simulink model "OneRobot_proporcional"  (R2021b)
settings: Solver=FixedStepDiscrete  StartTime=0.0  StopTime=t_sim  FixedStep=0.01  RelTol=1e-3  EnableMultiTasking=on
model workspace (MAT data in the model file):
  rampa = 1
values from neighbouring files (symbols this model uses):
  x = x-0.1    [movimiento.m]
  y = y-0.1    [movimiento.m]
undefined symbols (not defined in the file or in its folder): a, Angular, Linear, rx1, ry1
libraries: robotlib x4, robotcorelib x1, robotalgslib x1
settings Model: PacingRate=0.450000  Creator=The MathWorks, Inc.  LastModifiedBy=Cinthy
settings SolverCC: ConcurrentTasks=on  AlgebraicLoopSolver=TrustRegion  AutoInsertRateTranBlk=on
settings DataIOCC: LimitDataPoints=on  SaveFormat=StructureWithTime  ReturnWorkspaceOutputs=off
settings OptimizationCC: BlockReduction=off  EnhancedBackFolding=on  PassReuseOutputArgsAs=Individual arguments  ZeroExternalMemoryAtStartup=off  ZeroInternalMemoryAtStartup=off  MaxStackSize=64  OptimizeBlockOrder=speed  DifferentSizesBufferReuse=on  OptimizationCustomize=off  EfficientTunableParamExpr=on
settings DebuggingCC: SolverPrmCheckMsg=warning  ParameterTunabilityLossMsg=error  SFUnexpectedBacktrackingDiag=warning  SFNoUnconditionalDefaultTransitionDiag=warning  SFExecutionAtInitializationDiag=none  SFMachineParentedDataDiag=warning  ArithmeticOperatorsInVariantConditions=warning
settings HardwareCC: ProdBitPerPointer=32  ProdBitPerSizeT=32  ProdBitPerPtrDiffT=32  ProdLargestAtomicFloat=None  ProdIntDivRoundTo=Undefined  ProdEndianess=Unspecified  ProdWordSize=32  ProdHWDeviceType=Generic->Unspecified (assume 32-bit Generic)  TargetHWDeviceType=Generic->Unspecified (assume 32-bit Generic)
settings ModelReferenceCC: PropagateSignalLabelsOutOfModel=off
settings SFSimCC: SimUseLocalCustomCode=off  MATLABDynamicMemAlloc=off  CustomCodeUndefinedFunction=UseInterfaceOnly  SimTargetLang=C++
settings RTWCC: Description=Embedded Coder  SystemTargetFile=ert.tlc  HardwareBoard=Robot Operating System (ROS)  TLCOptions="-aInlineSetEventsForThisBaseRateFcn=TLC_FALSE -aSuppressMultiTaskScheduler=TLC_FALSE  -aRateBasedStepFcn=0"  TemplateMakefile=ert_default_tmf  RTWUseLocalCustomCode=off  Toolchain=Catkin  TargetLang=C++
settings CodeAppCC: ForceParamTrailComments=on  IgnoreCustomStorageClasses=off  OperatorAnnotations=on  SimulinkDataObjDesc=on  SFDataObjDesc=on  InsertBlockDesc=on
settings ConfigComp: CovMetricSettings=dw  CovSaveCumulativeToWorkspaceVar=on  CovSaveSingleToWorkspaceVar=on  CovExternalEMLEnable=off  CovSFcnEnable=off

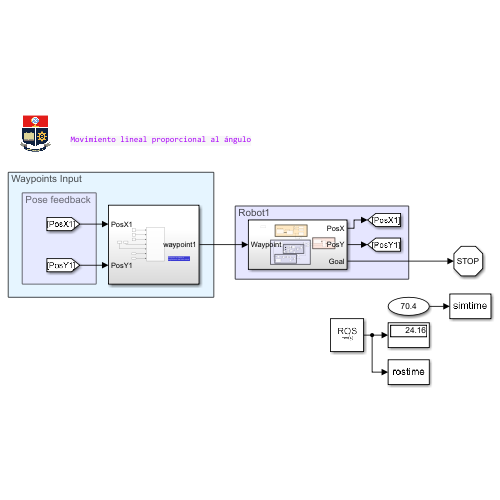
[thumbnail: Simulink's stored preview of the top-level diagram]
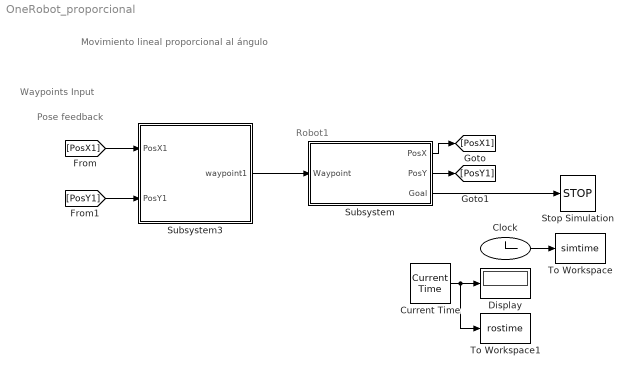
== system OneRobot_proporcional ==
  note: Movimiento lineal proporcional al ángulo
  note: Pose feedback
  note: Robot1
  note: Waypoints Input
  Clock : Clock
  Current Time : robotlib/Current Time  OutputFormat=double  SampleTime=-1  ModelName=OneRobot_proporcional
      settings: SourceProductBaseCode=RR
  Display : Display
  Stop Simulation : Stop
  Subsystem : Subsystem
  Subsystem3 : Subsystem
  To Workspace : ToWorkspace  VariableName=simtime  SampleTime=-1
  To Workspace1 : ToWorkspace  VariableName=rostime  SampleTime=-1
  wires:
  Subsystem/1(PosX) -> [PosX1]
  Subsystem/2(PosY) -> [PosY1]
  Subsystem3/1(waypoint1) -> Subsystem/1(Waypoint)
  Subsystem/3(Goal) -> Stop Simulation/1
  Clock/1 -> To Workspace/1
  [PosX1] -> Subsystem3/1(PosX1)
  [PosY1] -> Subsystem3/2(PosY1)
  Current Time/1 -> To Workspace1/1, Display/1

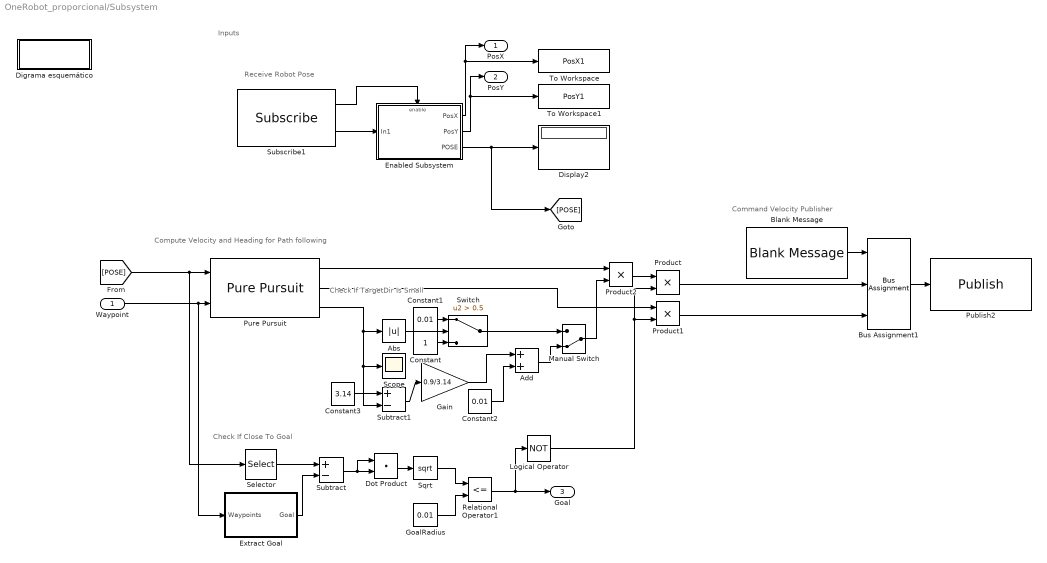
== system OneRobot_proporcional/Subsystem ==
  note: Check If TargetDir Is Small
  note: Compute Velocity and Heading for Path following
  note: Inputs
  note: Receive Robot Pose
  note: Check If Close To Goal
  note: Command Velocity Publisher
  Waypoint : Inport
  " Extract Goal" : MATLAB Function  TreatAsAtomicUnit=on
  Abs : Abs
  Add : Sum
  Blank Message : robotlib/Blank Message  messageClass=Message  entityType=geometry_msgs/Twist  messageType=geometry_msgs/Twist  SampleTime=inf  legacyBusStruct=off
  Bus Assignment1 : BusAssignment  DialogController=Simulink.DDGSource_BusAssignment  AssignedSignals=Linear.X,Angular.Z
  Constant : Constant
  Constant1 : Constant  Value=0.01
  Constant2 : Constant  Value=0.01
  Constant3 : Constant  Value=3.14
  Digrama esquemático : Subsystem
  Display2 : Display
  Dot Product : DotProduct  InputSameDT=on  OutDataTypeStr=Inherit: Inherit via internal rule
  Enabled Subsystem : Subsystem
  Gain : Gain  Gain=0.9/3.14
  GoalRadius : Constant  Value=0.01
  Logical Operator : Logic  Operator=NOT  AllPortsSameDT=off  OutDataTypeStr=boolean
  Manual Switch : ManualSwitch  CurrentSetting=0
  Product : Product
  Product1 : Product
  Product2 : Product
  Publish2 : robotlib/Publish  topicSource=Select from ROS network  topic=/robot1/cmd_vel  messageType=geometry_msgs/Twist  legacyBusStruct=off  messageQueueLength=105
  Pure Pursuit : robotalgslib/Pure Pursuit  DesiredLinearVelocity=0.22  MaxAngularVelocity=2.84  LookaheadDistance=1  TargetDirPort=on  SimulateUsing=Code generation
  Relational Operator1 : RelationalOperator  Operator=<=  OutDataTypeStr=boolean  RndMeth=Simplest
  Scope : Scope
  Selector : Selector  InputPortWidth=3  IndexOptions=Index vector (dialog)  Indices=[1 2]  OutputSizes=1
  Sqrt : Sqrt  SaturateOnIntegerOverflow=on
  Subscribe1 : robotlib/Subscribe  topicSource=Select from ROS network  topic=/robot1/odom  messageType=nav_msgs/Odometry  SampleTime=-1  legacyBusStruct=off  messageQueueLength=51
  Subtract : Sum  Inputs=+-
  Subtract1 : Sum  Inputs=+-
  Switch : Switch  Criteria=u2 > Threshold  Threshold=0.5
  To Workspace : ToWorkspace  VariableName=PosX1  SampleTime=-1
  To Workspace1 : ToWorkspace  VariableName=PosY1  SampleTime=-1
  PosX : Outport
  PosY : Outport  Port=2
  Goal : Outport  Port=3
  wires:
  GoalRadius/1 -> Relational Operator1/2
  Blank Message/1 -> Bus Assignment1/1
  Enabled Subsystem/3(POSE) -> [POSE], Display2/1
  Subtract/1 -> Dot Product/1, Dot Product/2
  Enabled Subsystem/2(PosY) -> PosY/1, To Workspace1/1
  Subscribe1/2 -> Enabled Subsystem/1(In1)
  Pure Pursuit/2 -> Product1/1
  Subscribe1/1 -> Enabled Subsystem/Enable
  Enabled Subsystem/1(PosX) -> PosX/1, To Workspace/1
  Relational Operator1/1 -> Logical Operator/1, Goal/1
  Product/1 -> Bus Assignment1/2
  Bus Assignment1/1 -> Publish2/1
  [POSE] -> Pure Pursuit/1, Selector/1
  Dot Product/1 -> Sqrt/1
  " Extract Goal"/1(Goal) -> Subtract/2
  Selector/1 -> Subtract/1
  Sqrt/1 -> Relational Operator1/1
  Logical Operator/1 -> Product1/2, Product/2
  Product1/1 -> Bus Assignment1/3
  Waypoint/1 -> " Extract Goal"/1(Waypoints), Pure Pursuit/2
  Pure Pursuit/3 -> Subtract1/2, Scope/1, Abs/1
  Constant/1 -> Switch/3
  Constant1/1 -> Switch/1
  Product2/1 -> Product/1
  Abs/1 -> Switch/2
  Pure Pursuit/1 -> Product2/1
  Constant2/1 -> Add/2
  Gain/1 -> Add/1
  Add/1 -> Manual Switch/2
  Manual Switch/1 -> Product2/2
  Switch/1 -> Manual Switch/1
  Constant3/1 -> Subtract1/1
  Subtract1/1 -> Gain/1

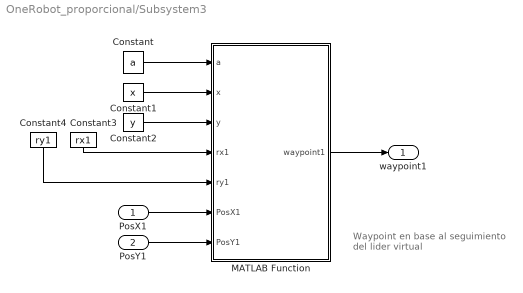
== system OneRobot_proporcional/Subsystem3 ==
  note: Waypoint en base al seguimiento del lider virtual
  PosX1 : Inport
  PosY1 : Inport  Port=2
  Constant : Constant  Value=a
  Constant1 : Constant  Value=x
  Constant2 : Constant  Value=y
  Constant3 : Constant  Value=rx1
  Constant4 : Constant  Value=ry1
  MATLAB Function : MATLAB Function  TreatAsAtomicUnit=on
  waypoint1 : Outport
  wires:
  Constant/1 -> MATLAB Function/1(a)
  Constant2/1 -> MATLAB Function/3(y)
  Constant1/1 -> MATLAB Function/2(x)
  PosX1/1 -> MATLAB Function/6(PosX1)
  MATLAB Function/1(waypoint1) -> waypoint1/1
  PosY1/1 -> MATLAB Function/7(PosY1)
  Constant3/1 -> MATLAB Function/4(rx1)
  Constant4/1 -> MATLAB Function/5(ry1)

== system OneRobot_proporcional/Subsystem/Digrama esquemático ==
  note: Definición de Velocidad lineal y angular
  note: >
  note: _____
  note: Waypoint
  note: |
      | |
      | |
  note: / |
      | [POSE] |
      | \_______|
  note: ______|
  note: Definir mensaje a enviar
  note: Comprobar si llegó a la meta
  note: Condiconamiento de Velocidad lineal
  note: Envio Velocidades al Robot
  note: Control Pure Pursuit
  note: Visualización
  note: Procesamiento de datos
  note: Recibir Pose del Robot
  note: | \
      | | [POSE]
      | |_______/
  note: >
  note: _____
  note: >
  note: _____
  note: _____
  note: >
  note: _____
  note: >
  note: _____
  note: >
  note: >
  note: _____
  note: >
  note: _____
  note: __________________
  note: >
  note: _____
  note: >
  note: _____
  note: >
  note: |
  note: >
  note: ____________________
  note: |
  note: >
  note: ___
  note: |
  note: |
  note: |
  note: ___
  note: _______________________________
  note: >
  note: ___
  note: |
  note: >
  note: _____
  note: |
  note: |
  note: |
  note: |
  note: |
  note: |
  note: |
  note: |
  note: |
  note: |
  note: |
  note: |
  note: |
  note: |
  note: |
  note: |

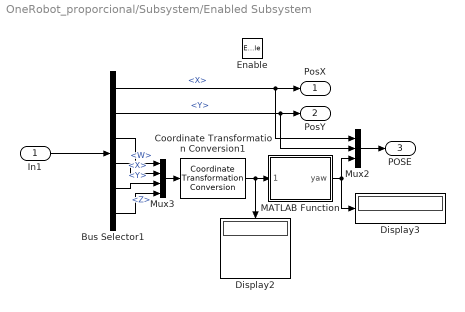
== system OneRobot_proporcional/Subsystem/Enabled Subsystem ==
  In1 : Inport
  Enable : EnablePort
  Bus Selector1 : BusSelector  DialogController=Simulink.DDGSource_BusSelector  OutputSignals=Pose.Pose.Position.X,Pose.Pose.Position.Y,Pose.Pose.Orientation.W,Pose.Pose.Orientation.X,Pose.Pose.Orientation.Y,Pose.Pose.Orientation.Z
  Coordinate Transformation Conversion1 : robotcorelib/Coordinate Transformation Conversion  InputRepresentation=Quaternion  InputEulerSequence=ZYX  ShowTrVecInputPort=on  OutputRepresentation=Euler Angles  OutputEulerSequence=ZYX  ShowTrVecOutputPort=on  SimulateUsing=Interpreted execution
      settings: SourceProductBaseCode=NV,RO,RR,UV
  Display2 : Display
  Display3 : Display
  MATLAB Function : MATLAB Function  TreatAsAtomicUnit=on
  Mux2 : Mux  Inputs=3
  Mux3 : Mux
  PosX : Outport  VectorParamsAs1DForOutWhenUnconnected=off
  PosY : Outport  Port=2  VectorParamsAs1DForOutWhenUnconnected=off
  POSE : Outport  Port=3
  wires:
  Bus Selector1/5 -> Mux3/3  "<Y>"
  Bus Selector1/1 -> PosX/1, Mux2/1  "<X>"
  Bus Selector1/3 -> Mux3/1  "<W>"
  Mux2/1 -> POSE/1
  In1/1 -> Bus Selector1/1
  Coordinate Transformation Conversion1/1 -> Display2/1, MATLAB Function/1(eulerAng)
  Bus Selector1/4 -> Mux3/2  "<X>"
  Bus Selector1/6 -> Mux3/4  "<Z>"
  MATLAB Function/1(yaw) -> Mux2/3, Display3/1
  Bus Selector1/2 -> PosY/1, Mux2/2  "<Y>"
  Mux3/1 -> Coordinate Transformation Conversion1/1

== matlab function OneRobot_proporcional/Subsystem/Enabled Subsystem/MATLAB Function ==
  data: eulerAng input; yaw output
function yaw = fcn(eulerAng)

yaw = eulerAng(1);

== matlab function OneRobot_proporcional/Subsystem3/MATLAB Function ==
  data: a input; x input; y input; rx1 input; ry1 input; waypoint1 output; PosX1 input; PosY1 input
function waypoint1 = waypoint_metod(a, x, y, rx1, ry1, PosX1, PosY1)

if a==2||a==3||a==4 %no importa el metodo ya que es solo un agente
    waypoint1=[PosX1(length(PosX1)) PosY1(length(PosY1));x+rx1 y+ry1];
%     waypoint2=[PosX2(length(PosX2)) PosY2(length(PosY2));x+rx2 y+ry2];
%     waypoint3=[PosX3(length(PosX3)) PosY3(length(PosY3));x+rx3 y+ry3];
% elseif a==4
%     waypoint1=[PosX1(length(PosX1)) PosY1(length(PosY1));PosX2(length(PosX2))+rx1-rx2 PosY2(length(PosY2))+ry1-ry2];
%     waypoint2=[PosX2(length(PosX2)) PosY2(length(PosY2));x+rx2 y+ry2];
%     waypoint3=[PosX3(length(PosX3)) PosY3(length(PosY3));PosX2(length(PosX2))+rx3-rx2 PosY2(length(PosY2))+ry3-ry2];  
else
    waypoint1=[PosX1(length(PosX1)) PosY1(length(PosY1));PosX1(length(PosX1)) PosY1(length(PosY1))];
%     waypoint2=[PosX2(length(PosX2)) PosY2(length(PosY2));PosX2(length(PosX2)) PosY2(length(PosY2))];
%     waypoint3=[PosX3(length(PosX3)) PosY3(length(PosY3));PosX3(length(PosX3)) PosY3(length(PosY3))];
end

== matlab function OneRobot_proporcional/Subsystem/ Extract Goal ==
  data: Waypoints input; Goal output
function Goal = extractGoal(Waypoints)
%#codegen
b = isnan(Waypoints);
[rows,~] = find(b);
ridx = setdiff(1:size(Waypoints,1), sort(rows));
Goal = [Waypoints(ridx(end), 1) Waypoints(ridx(end), 2)];
